simulink model "cichbcic_core"  (Simulink 7.9)
settings: Solver=ode45  StartTime=0.0  StopTime=10.0  RelTol=1e-3
libraries: xbsIndex_r4 x375
(part 1 of 5)
settings Model: Creator=chenhong  LastModifiedBy=chenhong

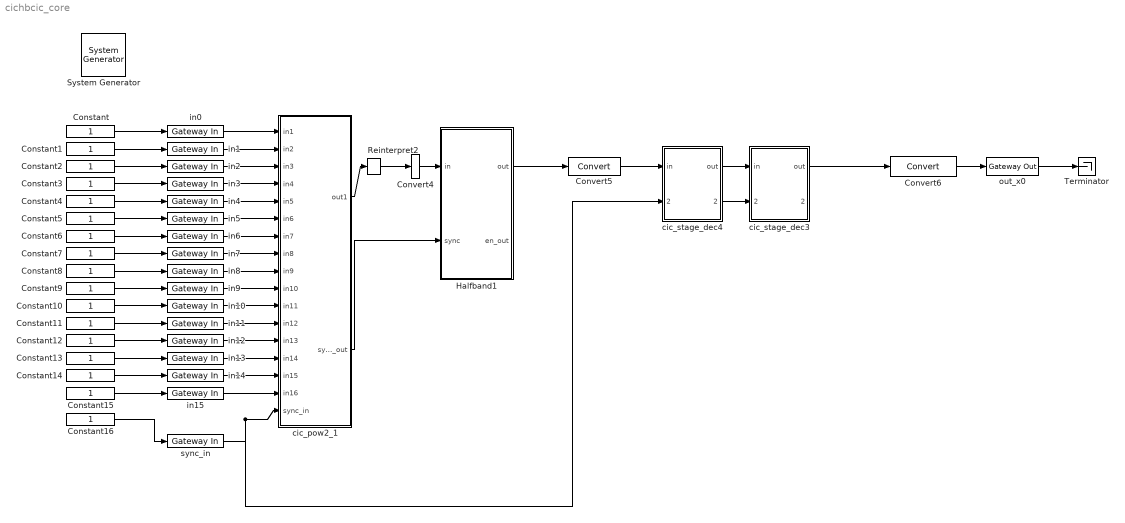
== system cichbcic_core ==
  " System Generator" : xbsIndex_r4/ System Generator  Tag=genX  xilinxfamily=virtex6  part=xc6vsx475t  speed=-1  package=ff1759  synthesis_tool=XST  clock_wrapper=Clock Enables  directory=./cichbcic_core  proj_type=Project Navigator  Synth_file=XST Defaults  Impl_file=ISE Defaults  testbench=off  simulink_period=1  sysclk_period=6.6667  dcm_input_clock_period=100  incr_netlist=off  trim_vbits=Everywhere in SubSystem  dbl_ovrd=According to Block Masks  core_generation=According to Block Masks  run_coregen=off  deprecated_control=off  eval_field=0  block_type=sysgen
  Constant{,1..16} (17 alike) : Constant
  Convert4 : xbsIndex_r4/Convert  gui_display_data_type=Fixed-point  arith_type="Signed  (2's comp)"  n_bits=32  bin_pt=18  float_type=Single  exp_bits=8  fraction_bits=24  quantization=Truncate  overflow=Wrap  en=off  latency=1  dbl_ovrd=off  pipeline=off  block_type=convert
  Convert5 : xbsIndex_r4/Convert  gui_display_data_type=Fixed-point  arith_type="Signed  (2's comp)"  n_bits=32  bin_pt=12  float_type=Single  exp_bits=8  fraction_bits=24  quantization=Truncate  overflow=Wrap  en=off  latency=1  dbl_ovrd=off  pipeline=off  block_type=convert
  Convert6 : xbsIndex_r4/Convert  gui_display_data_type=Fixed-point  arith_type="Signed  (2's comp)"  n_bits=32  bin_pt=6  float_type=Single  exp_bits=8  fraction_bits=24  quantization=Truncate  overflow=Wrap  en=off  latency=1  dbl_ovrd=off  pipeline=off  block_type=convert
  Halfband1 : Subsystem  AncestorBlock=gbt_library/Halfband  mask(Halfband FIR){mult_latency=3, add_latency=2, hold_period=2, passband=0.4, fir_len=7}
      mask prompts: mult_latency "Multiplication latency"; add_latency "Add latency"; hold_period "Hold Period"; passband "Width of Halfband passband (<0.5)"; fir_len "FIR Length (odd) [Number of Taps will be: 2*fir_len+1]"
      mask help: A halfband FIR for low rate computation.
      mask init:
      | coeffs = halfband_coeff_gen(fir_len, passband);
      | config.source=str2func('hold_fir_init_xblock');
      | config.depend=[get_dependlist('hold_fir'),{'halfband_coeff_gen'}];
      | config.toplevel=gcb;
      | set_param(gcb,'LinkStatus','inactive');
      | xBlock(config, {config.toplevel,...
      |     'mult_latency', mult_latency, ...
      |     'add_latency', add_latency, ...
      |     'hold_period', hold_period, ...
      |     'coeffs', coeffs});
      settings: AttributesFormatString=|
      | 15-tap FIR filter (9 nonzero tap)
      |  hold period: 2
      |  mult latency: 3
      |  add latency: 2
  Reinterpret2 : xbsIndex_r4/Reinterpret  force_arith_type=off  arith_type="Signed  (2's comp)"  force_bin_pt=on  bin_pt=30  block_type=reinterpret
  Terminator : Terminator
  cic_pow2_1 : Subsystem  AncestorBlock=gbt_library/cic_pow2  mask(CIC (pow2)){n_stages=4, dec_rate=32, input_clk_period=1, n_inputs=16, add_latency=1, n_bits=24, bin_pt=22}
      mask prompts: n_stages "CIC filter Order"; dec_rate "Decimation rate"; input_clk_period "Input Clock Period"; n_inputs "Number of inputs"; add_latency "Add latency"; n_bits "Input bit width"; bin_pt "Binary point"
      mask help:
      | A non-recursive CIC filter with parallel inputs.
      | Supports decimation rate of power of 2.
      | A multi-stage implementation with each stage of decimation rate 2.
      mask init:
      | config.source = str2func('cic_pow2_init_xblock');
      | config.toplevel = gcb;
      | config.depend = get_dependlist('cic_pow2'); 
      | set_param(gcb,'LinkStatus','inactive');
      | xBlock(config, {config.toplevel,...
      |                 'n_stages',n_stages, ...
      |                 'dec_rate', dec_rate, ...
      |                 'input_clk_rate', input_clk_period, ...
      |                 'n_inputs', n_inputs,...
      |                 'add_latency',add_latency,...
      |                 'n_bits', n_bits, ...
      |                 'bin_pt', bin_pt} ...
      |                 );
      | disp('new block added');
      settings: AttributesFormatString=|
      | dec_rate = 32
      | Order = 4
  cic_stage_dec3 : Subsystem  AncestorBlock=gbt_library/cic_stage_dec2  mask(CIC stage (dec2)){n_stages=3, recursive=off, dec_rate=2, n_inputs=1, input_clk_period=1, input_period=4, add_latency=2, n_bits=35, bin_pt=12}
      mask prompts: n_stages "CIC filter Order"; recursive "Recursive?"; dec_rate "Decimation rate"; n_inputs "Number of Inputs"; input_clk_period "Input Clock period (Actual)"; input_period "Effective Input Sampling Period"; add_latency "Add latency"; n_bits "Input bit width"; bin_pt "Binary point"
      mask help:
      | A single stage of CIC filter with even number of parallel inputs.
      | Only supports decimation rate = 2.
      | If n_inputs > 1, number of outputs = n_inputs/2.
      | Non-recursive.
      |
      | Clock period:
      | input_clk_period is the actual sampling period of incoming data stream.
      | input_period is the effective (or expected) sampling period of incoming data stream.
      | E.g. For incoming data stream X[n] = [1& 1 2 2 3 3 4 4 5 5 ...], the input_clk_period is 1 and the input_period is 2.
      mask init:
      | if recursive
      |     % recursive case
      |     config.source=str2func('cic_stage_dec2_recursive_init_xblock');
      |     config.toplevel=gcb;
      |     config.depend = get_dependlist('cic_stage_dec2_recursive');
      |     set_param(gcb,'LinkStatus','inactive');
      |     xBlock(config, {config.toplevel, ...
      |                 'n_stages', n_stages, ...
      |                 'dec_rate', dec_rate, ...
      |                 'n_inputs', n_inputs, ...
      |                 'input_clk_period', input_clk_period, ...
      |                 'input_period', input_period, ...
      |                 'add_latency', add_latency, ...
      |                 'input_bits', n_bits, ...
      |                 'bin_pt', bin_pt, ...
      |                 'delay_len', 1});
      | else
      |     % non-recursive case
      |     config.source=str2func('cic_stage_dec2_init_xblock');
      |     config.toplevel=gcb;
      |     config.depend = get_dependlist('cic_stage_dec2');
      |     set_param(gcb,'LinkStatus','inactive');
      |     xBlock(config, {config.toplevel, ...
      |                 'n_stages', n_stages, ...
      |                 'dec_rate', dec_rate, ...
      |                 'n_inputs', n_inputs, ...
      |                 'input_clk_period', input_clk_period, ...
      |                 'input_period', input_period, ...
      |                 'add_latency', add_latency, ...
      |                 'n_bits', n_bits, ...
      |                 'bin_pt', bin_pt});
      | end
      settings: AttributesFormatString=|
      | nonrecursive
      | 35_12_in
      | clock(actualy/effective): 1/4
      mask CallbackString:
      | ||n=get_param(gcb,'dec_rate');
      | if ~isempty(n)
      |     n = eval(n);
      |     if ~isprime(n) && n~=1
      |         errordlg('Only supports decimation rate that is a prime number or 1');
      |         set_param(gcb,'dec_rate','');
      |     end
      | end||||||
  cic_stage_dec4 : Subsystem  AncestorBlock=gbt_library/cic_stage_dec2  mask(CIC stage (dec2)){n_stages=3, recursive=off, dec_rate=2, n_inputs=1, input_clk_period=1, input_period=2, add_latency=2, n_bits=32, bin_pt=12}
      mask prompts: n_stages "CIC filter Order"; recursive "Recursive?"; dec_rate "Decimation rate"; n_inputs "Number of Inputs"; input_clk_period "Input Clock period (Actual)"; input_period "Effective Input Sampling Period"; add_latency "Add latency"; n_bits "Input bit width"; bin_pt "Binary point"
      mask help:
      | A single stage of CIC filter with even number of parallel inputs.
      | Only supports decimation rate = 2.
      | If n_inputs > 1, number of outputs = n_inputs/2.
      | Non-recursive.
      |
      | Clock period:
      | input_clk_period is the actual sampling period of incoming data stream.
      | input_period is the effective (or expected) sampling period of incoming data stream.
      | E.g. For incoming data stream X[n] = [1& 1 2 2 3 3 4 4 5 5 ...], the input_clk_period is 1 and the input_period is 2.
      mask init: same as cichbcic_core/cic_stage_dec3
      settings: AttributesFormatString=|
      | nonrecursive
      | 32_12_in
      | clock(actualy/effective): 1/2
      mask CallbackString:
      | ||n=get_param(gcb,'dec_rate');
      | if ~isempty(n)
      |     n = eval(n);
      |     if ~isprime(n) && n~=1
      |         errordlg('Only supports decimation rate that is a prime number or 1');
      |         set_param(gcb,'dec_rate','');
      |     end
      | end||||||
  in{0..15} (16 alike) : xbsIndex_r4/Gateway In  gui_display_data_type=Fixed-point  arith_type="Signed  (2's comp)"  n_bits=24  bin_pt=22  preci_type=Single  exp_width=8  frac_width=24  quantization="Round  (unbiased: +/- Inf)"  overflow=Saturate  period=1  dbl_ovrd=off  timing_constraint=None  locs_specified=off  LOCs={}  UseAsADC=off  ADCChannel='1'  inherit_from_input=off  hdl_port=on  block_type=gatewayin
  out_x0 : xbsIndex_r4/Gateway Out  inherit_from_input=off  hdl_port=on  timing_constraint=None  locs_specified=off  LOCs={}  UseAsDAC=off  DACChannel='1'  block_type=gatewayout
  sync_in : xbsIndex_r4/Gateway In  gui_display_data_type=Boolean  arith_type=Boolean  n_bits=24  bin_pt=22  preci_type=Single  exp_width=8  frac_width=24  quantization="Round  (unbiased: +/- Inf)"  overflow=Saturate  period=1  dbl_ovrd=off  timing_constraint=None  locs_specified=off  LOCs={}  UseAsADC=off  ADCChannel='1'  inherit_from_input=off  hdl_port=on  block_type=gatewayin
  wires:
  cic_stage_dec4/2(sync_out) -> cic_stage_dec3/2(sync_in)
  cic_stage_dec4/1(out) -> cic_stage_dec3/1(in)
  Halfband1/1(out) -> Convert5/1
  cic_pow2_1/1(out1) -> Reinterpret2/1
  cic_pow2_1/2(sync_out) -> Halfband1/2(sync)
  Convert4/1 -> Halfband1/1(in)
  Convert5/1 -> cic_stage_dec4/1(in)
  Convert6/1 -> out_x0/1
  cic_stage_dec3/1(out) -> Convert6/1
  Reinterpret2/1 -> Convert4/1
  in0/1 -> cic_pow2_1/1(in1)
  in1/1 -> cic_pow2_1/2(in2)
  in2/1 -> cic_pow2_1/3(in3)
  in3/1 -> cic_pow2_1/4(in4)
  in4/1 -> cic_pow2_1/5(in5)
  in5/1 -> cic_pow2_1/6(in6)
  in6/1 -> cic_pow2_1/7(in7)
  in7/1 -> cic_pow2_1/8(in8)
  in8/1 -> cic_pow2_1/9(in9)
  in9/1 -> cic_pow2_1/10(in10)
  in10/1 -> cic_pow2_1/11(in11)
  in11/1 -> cic_pow2_1/12(in12)
  in12/1 -> cic_pow2_1/13(in13)
  in13/1 -> cic_pow2_1/14(in14)
  in14/1 -> cic_pow2_1/15(in15)
  in15/1 -> cic_pow2_1/16(in16)
  sync_in/1 -> cic_pow2_1/17(sync_in), cic_stage_dec4/2(sync_in)
  Constant/1 -> in0/1
  Constant1/1 -> in1/1
  Constant2/1 -> in2/1
  Constant3/1 -> in3/1
  Constant4/1 -> in4/1
  Constant5/1 -> in5/1
  Constant6/1 -> in6/1
  Constant7/1 -> in7/1
  Constant8/1 -> in8/1
  Constant9/1 -> in9/1
  Constant10/1 -> in10/1
  Constant11/1 -> in11/1
  Constant12/1 -> in12/1
  Constant13/1 -> in13/1
  Constant14/1 -> in14/1
  Constant15/1 -> in15/1
  Constant16/1 -> sync_in/1
  out_x0/1 -> Terminator/1

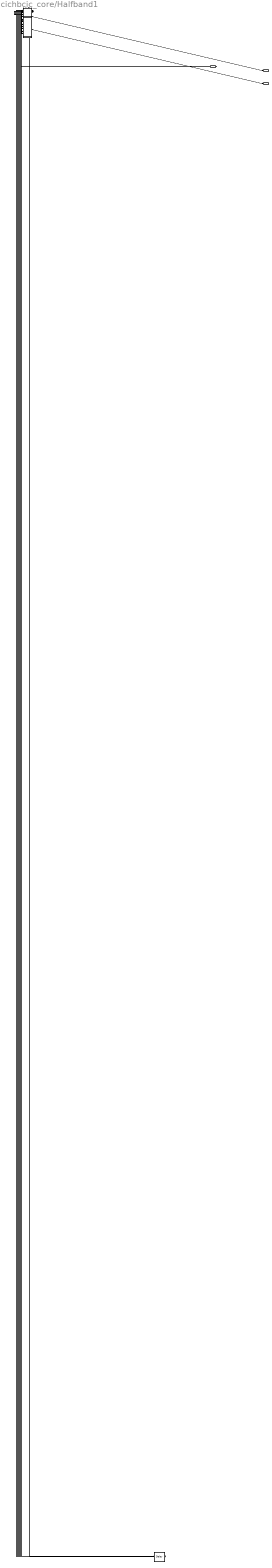
== system cichbcic_core/Halfband1 ==
  in : Inport
  sync : Inport  Port=2
  Delay{1..14} (14 alike) : xbsIndex_r4/Delay  rst=off  infoeditControl=Selection of Reset will increase slice count due to use of real FFs and instead of SRLs  en=off  latency=2  dbl_ovrd=off  reg_retiming=off  block_type=delay
  adder_tree : Subsystem
      settings: AttributesFormatString=|
      | latency 8
      | hold period:2
  en_gen : Subsystem
      settings: AttributesFormatString=|
      | hold period: 2
      | explicit clk period:off , input clk period:1
  hold_fir_tap1 : Subsystem
      settings: AttributesFormatString=|
      | coefficient: -0.026473
      |  hold period: 2
      |  mult latency: 3
  hold_fir_tap11 : Subsystem
      settings: AttributesFormatString=|
      | coefficient: -0.093407
      |  hold period: 2
      |  mult latency: 3
  hold_fir_tap13 : Subsystem
      settings: AttributesFormatString=|
      | coefficient: 0.044090
      |  hold period: 2
      |  mult latency: 3
  hold_fir_tap15 : Subsystem
      settings: AttributesFormatString=|
      | coefficient: -0.026473
      |  hold period: 2
      |  mult latency: 3
  hold_fir_tap3 : Subsystem
      settings: AttributesFormatString=|
      | coefficient: 0.044090
      |  hold period: 2
      |  mult latency: 3
  hold_fir_tap5 : Subsystem
      settings: AttributesFormatString=|
      | coefficient: -0.093407
      |  hold period: 2
      |  mult latency: 3
  hold_fir_tap7 : Subsystem
      settings: AttributesFormatString=|
      | coefficient: 0.313910
      |  hold period: 2
      |  mult latency: 3
  hold_fir_tap8 : Subsystem
      settings: AttributesFormatString=|
      | coefficient: 0.500000
      |  hold period: 2
      |  mult latency: 3
  hold_fir_tap9 : Subsystem
      settings: AttributesFormatString=|
      | coefficient: 0.313910
      |  hold period: 2
      |  mult latency: 3
  out : Outport
  en_out : Outport  Port=2
  wires:
  sync/1 -> en_gen/1(sync_in)
  in/1 -> Delay1/1, hold_fir_tap1/1(data_in)
  Delay1/1 -> Delay2/1  "xlsub2_Delay_out1"
  Delay2/1 -> Delay3/1, hold_fir_tap3/1(data_in)  "xlsub2_Delay_out2"
  Delay3/1 -> Delay4/1  "xlsub2_Delay_out3"
  Delay4/1 -> Delay5/1, hold_fir_tap5/1(data_in)  "xlsub2_Delay_out4"
  Delay5/1 -> Delay6/1  "xlsub2_Delay_out5"
  Delay6/1 -> Delay7/1, hold_fir_tap7/1(data_in)  "xlsub2_Delay_out6"
  Delay7/1 -> Delay8/1, hold_fir_tap8/1(data_in)  "xlsub2_Delay_out7"
  Delay8/1 -> Delay9/1, hold_fir_tap9/1(data_in)  "xlsub2_Delay_out8"
  Delay9/1 -> Delay10/1  "xlsub2_Delay_out9"
  Delay10/1 -> Delay11/1, hold_fir_tap11/1(data_in)  "xlsub2_Delay_out10"
  Delay11/1 -> Delay12/1  "xlsub2_Delay_out11"
  Delay12/1 -> Delay13/1, hold_fir_tap13/1(data_in)  "xlsub2_Delay_out12"
  Delay13/1 -> Delay14/1  "xlsub2_Delay_out13"
  en_gen/1(en_out) -> hold_fir_tap1/2(en_in), hold_fir_tap3/2(en_in), hold_fir_tap5/2(en_in), hold_fir_tap7/2(en_in), hold_fir_tap8/2(en_in), hold_fir_tap9/2(en_in), hold_fir_tap11/2(en_in), hold_fir_tap13/2(en_in), hold_fir_tap15/2(en_in), adder_tree/1(en_in)  "en"
  Delay14/1 -> hold_fir_tap15/1(data_in)  "xlsub2_Delay_out14"
  hold_fir_tap1/1(mult_out) -> adder_tree/2(din1)  "hold_fir_tap_out1"
  hold_fir_tap3/1(mult_out) -> adder_tree/3(din2)  "hold_fir_tap_out2"
  hold_fir_tap5/1(mult_out) -> adder_tree/4(din3)  "hold_fir_tap_out3"
  hold_fir_tap7/1(mult_out) -> adder_tree/5(din4)  "hold_fir_tap_out4"
  hold_fir_tap8/1(mult_out) -> adder_tree/6(din5)  "hold_fir_tap_out5"
  hold_fir_tap9/1(mult_out) -> adder_tree/7(din6)  "hold_fir_tap_out6"
  hold_fir_tap11/1(mult_out) -> adder_tree/8(din7)  "hold_fir_tap_out7"
  hold_fir_tap13/1(mult_out) -> adder_tree/9(din8)  "hold_fir_tap_out8"
  hold_fir_tap15/1(mult_out) -> adder_tree/10(din9)  "hold_fir_tap_out9"
  adder_tree/1(en_out) -> en_out/1
  adder_tree/2(dout) -> out/1

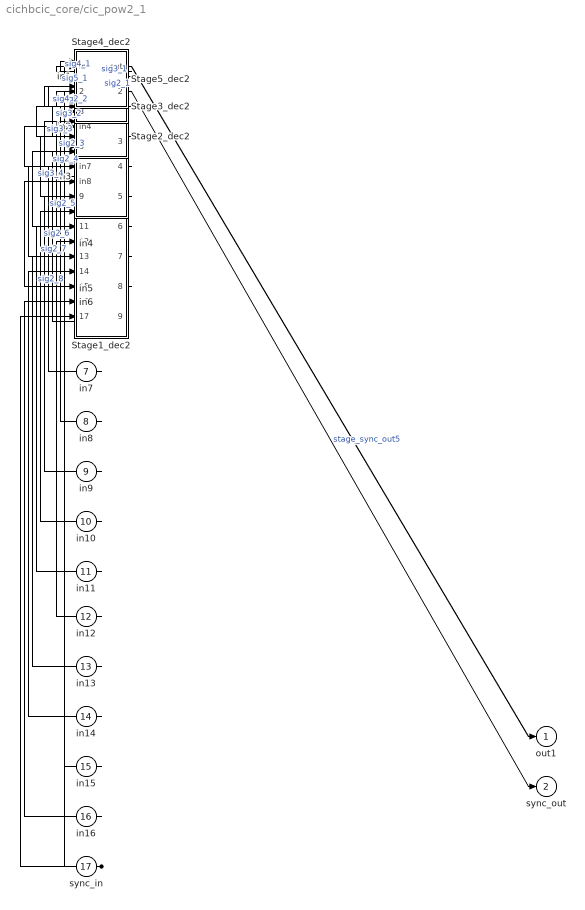
== system cichbcic_core/cic_pow2_1 ==
  in1 : Inport
  in2 : Inport  Port=2
  in3 : Inport  Port=3
  in4 : Inport  Port=4
  in5 : Inport  Port=5
  in6 : Inport  Port=6
  in7 : Inport  Port=7
  in8 : Inport  Port=8
  in9 : Inport  Port=9
  in10 : Inport  Port=10
  in11 : Inport  Port=11
  in12 : Inport  Port=12
  in13 : Inport  Port=13
  in14 : Inport  Port=14
  in15 : Inport  Port=15
  in16 : Inport  Port=16
  sync_in : Inport  Port=17
  Stage1_dec2 : Subsystem
      settings: AttributesFormatString=|
      | nonrecursive
      | 24_22_in
      | clock(actualy/effective): 1/1
  Stage2_dec2 : Subsystem
      settings: AttributesFormatString=|
      | nonrecursive
      | 28_22_in
      | clock(actualy/effective): 1/1
  Stage3_dec2 : Subsystem
      settings: AttributesFormatString=|
      | nonrecursive
      | 32_22_in
      | clock(actualy/effective): 1/1
  Stage4_dec2 : Subsystem
      settings: AttributesFormatString=|
      | nonrecursive
      | 36_22_in
      | clock(actualy/effective): 1/1
  Stage5_dec2 : Subsystem
      settings: AttributesFormatString=|
      | nonrecursive
      | 40_22_in
      | clock(actualy/effective): 1/1
  out1 : Outport
  sync_out : Outport  Port=2
  wires:
  in1/1 -> Stage1_dec2/1(in1)
  in2/1 -> Stage1_dec2/2(in2)
  in3/1 -> Stage1_dec2/3(in3)
  in4/1 -> Stage1_dec2/4(in4)
  in5/1 -> Stage1_dec2/5(in5)
  in6/1 -> Stage1_dec2/6(in6)
  in7/1 -> Stage1_dec2/7(in7)
  in8/1 -> Stage1_dec2/8(in8)
  in9/1 -> Stage1_dec2/9(in9)
  in10/1 -> Stage1_dec2/10(in10)
  in11/1 -> Stage1_dec2/11(in11)
  in12/1 -> Stage1_dec2/12(in12)
  in13/1 -> Stage1_dec2/13(in13)
  in14/1 -> Stage1_dec2/14(in14)
  in15/1 -> Stage1_dec2/15(in15)
  in16/1 -> Stage1_dec2/16(in16)
  sync_in/1 -> Stage1_dec2/17(sync_in), Stage2_dec2/9(sync_in), Stage3_dec2/5(sync_in), Stage4_dec2/3(sync_in), Stage5_dec2/2(sync_in)
  Stage1_dec2/1(out1) -> Stage2_dec2/1(in1)  "sig2_1"
  Stage1_dec2/2(out2) -> Stage2_dec2/2(in2)  "sig2_2"
  Stage1_dec2/3(out3) -> Stage2_dec2/3(in3)  "sig2_3"
  Stage1_dec2/4(out4) -> Stage2_dec2/4(in4)  "sig2_4"
  Stage1_dec2/5(out5) -> Stage2_dec2/5(in5)  "sig2_5"
  Stage1_dec2/6(out6) -> Stage2_dec2/6(in6)  "sig2_6"
  Stage1_dec2/7(out7) -> Stage2_dec2/7(in7)  "sig2_7"
  Stage1_dec2/8(out8) -> Stage2_dec2/8(in8)  "sig2_8"
  Stage2_dec2/1(out1) -> Stage3_dec2/1(in1)  "sig3_1"
  Stage2_dec2/2(out2) -> Stage3_dec2/2(in2)  "sig3_2"
  Stage2_dec2/3(out3) -> Stage3_dec2/3(in3)  "sig3_3"
  Stage2_dec2/4(out4) -> Stage3_dec2/4(in4)  "sig3_4"
  Stage3_dec2/1(out1) -> Stage4_dec2/1(in1)  "sig4_1"
  Stage3_dec2/2(out2) -> Stage4_dec2/2(in2)  "sig4_2"
  Stage4_dec2/1(out1) -> Stage5_dec2/1(in)  "sig5_1"
  Stage5_dec2/1(out) -> out1/1
  Stage5_dec2/2(sync_out) -> sync_out/1  "stage_sync_out5"

== system cichbcic_core/cic_stage_dec3 ==
  in : Inport
  sync_in : Inport  Port=2
  Down_sample1 : Subsystem
      settings: AttributesFormatString=|
      | Rate change: 2
      | clock(actualy/effective): 1/4
  adder_tree1 : Subsystem
  adder_tree2 : Subsystem
  adder_tree3 : Subsystem
  delay1_1 : xbsIndex_r4/Delay  rst=off  infoeditControl=Selection of Reset will increase slice count due to use of real FFs and instead of SRLs  en=off  latency=4  dbl_ovrd=off  reg_retiming=off  block_type=delay
  delay2_1 : xbsIndex_r4/Delay  rst=off  infoeditControl=Selection of Reset will increase slice count due to use of real FFs and instead of SRLs  en=off  latency=4  dbl_ovrd=off  reg_retiming=off  block_type=delay
  delay3_1 : xbsIndex_r4/Delay  rst=off  infoeditControl=Selection of Reset will increase slice count due to use of real FFs and instead of SRLs  en=off  latency=4  dbl_ovrd=off  reg_retiming=off  block_type=delay
  out : Outport
  sync_out : Outport  Port=2
  wires:
  in/1 -> delay1_1/1, adder_tree1/1(sync), adder_tree1/2(din_1)
  delay1_1/1 -> adder_tree1/3(din_2)  "delay_out1_2"
  adder_tree1/2(dout) -> delay2_1/1, adder_tree2/2(din_1)  "delay_in1_1"
  adder_tree1/1(sync_out) -> adder_tree2/1(sync)  "adder_tree_sync_in2"
  delay2_1/1 -> adder_tree2/3(din_2)  "delay_out2_2"
  adder_tree2/2(dout) -> delay3_1/1, adder_tree3/2(din_1)  "delay_in2_1"
  adder_tree2/1(sync_out) -> adder_tree3/1(sync)  "adder_tree_sync_in3"
  delay3_1/1 -> adder_tree3/3(din_2)  "delay_out3_2"
  adder_tree3/2(dout) -> Down_sample1/1(In)  "delay_in3_1"
  sync_in/1 -> Down_sample1/2(sync_in)
  Down_sample1/1(Out) -> out/1
  Down_sample1/2(sync_out) -> sync_out/1

== system cichbcic_core/cic_stage_dec4 ==
  in : Inport
  sync_in : Inport  Port=2
  Down_sample1 : Subsystem
      settings: AttributesFormatString=|
      | Rate change: 2
      | clock(actualy/effective): 1/2
  adder_tree1 : Subsystem
  adder_tree2 : Subsystem
  adder_tree3 : Subsystem
  delay1_1 : xbsIndex_r4/Delay  rst=off  infoeditControl=Selection of Reset will increase slice count due to use of real FFs and instead of SRLs  en=off  latency=2  dbl_ovrd=off  reg_retiming=off  block_type=delay
  delay2_1 : xbsIndex_r4/Delay  rst=off  infoeditControl=Selection of Reset will increase slice count due to use of real FFs and instead of SRLs  en=off  latency=2  dbl_ovrd=off  reg_retiming=off  block_type=delay
  delay3_1 : xbsIndex_r4/Delay  rst=off  infoeditControl=Selection of Reset will increase slice count due to use of real FFs and instead of SRLs  en=off  latency=2  dbl_ovrd=off  reg_retiming=off  block_type=delay
  out : Outport
  sync_out : Outport  Port=2
  wires:
  in/1 -> delay1_1/1, adder_tree1/1(sync), adder_tree1/2(din_1)
  delay1_1/1 -> adder_tree1/3(din_2)  "delay_out1_2"
  adder_tree1/2(dout) -> delay2_1/1, adder_tree2/2(din_1)  "delay_in1_1"
  adder_tree1/1(sync_out) -> adder_tree2/1(sync)  "adder_tree_sync_in2"
  delay2_1/1 -> adder_tree2/3(din_2)  "delay_out2_2"
  adder_tree2/2(dout) -> delay3_1/1, adder_tree3/2(din_1)  "delay_in2_1"
  adder_tree2/1(sync_out) -> adder_tree3/1(sync)  "adder_tree_sync_in3"
  delay3_1/1 -> adder_tree3/3(din_2)  "delay_out3_2"
  adder_tree3/2(dout) -> Down_sample1/1(In)  "delay_in3_1"
  sync_in/1 -> Down_sample1/2(sync_in)
  Down_sample1/1(Out) -> out/1
  Down_sample1/2(sync_out) -> sync_out/1

== system cichbcic_core/Halfband1/adder_tree ==
  en_in : Inport
  din1 : Inport  Port=2
  din2 : Inport  Port=3
  din3 : Inport  Port=4
  din4 : Inport  Port=5
  din5 : Inport  Port=6
  din6 : Inport  Port=7
  din7 : Inport  Port=8
  din8 : Inport  Port=9
  din9 : Inport  Port=10
  addr1 : Subsystem
      settings: AttributesFormatString=|
      | hold period: 2
      |  add latency: 2
  addr11 : Subsystem
      settings: AttributesFormatString=|
      | hold period: 2
      |  add latency: 2
  addr2 : Subsystem
      settings: AttributesFormatString=|
      | hold period: 2
      |  add latency: 2
  addr3 : Subsystem
      settings: AttributesFormatString=|
      | hold period: 2
      |  add latency: 2
  addr4 : Subsystem
      settings: AttributesFormatString=|
      | hold period: 2
      |  add latency: 2
  addr6 : Subsystem
      settings: AttributesFormatString=|
      | hold period: 2
      |  add latency: 2
  addr7 : Subsystem
      settings: AttributesFormatString=|
      | hold period: 2
      |  add latency: 2
  addr9 : Subsystem
      settings: AttributesFormatString=|
      | hold period: 2
      |  add latency: 2
  dly10 : xbsIndex_r4/Delay  rst=off  infoeditControl=Selection of Reset will increase slice count due to use of real FFs and instead of SRLs  en=off  latency=4  dbl_ovrd=off  reg_retiming=on  block_type=delay
  dly5 : xbsIndex_r4/Delay  rst=off  infoeditControl=Selection of Reset will increase slice count due to use of real FFs and instead of SRLs  en=off  latency=4  dbl_ovrd=off  reg_retiming=on  block_type=delay
  dly8 : xbsIndex_r4/Delay  rst=off  infoeditControl=Selection of Reset will increase slice count due to use of real FFs and instead of SRLs  en=off  latency=4  dbl_ovrd=off  reg_retiming=on  block_type=delay
  sync_delay : xbsIndex_r4/Delay  rst=off  infoeditControl=Selection of Reset will increase slice count due to use of real FFs and instead of SRLs  en=off  latency=8  dbl_ovrd=off  reg_retiming=on  block_type=delay
  en_out : Outport
  dout : Outport  Port=2
  wires:
  en_in/1 -> sync_delay/1, addr1/3(en_in), addr2/3(en_in), addr3/3(en_in), addr4/3(en_in), addr6/3(en_in), addr7/3(en_in), addr9/3(en_in), addr11/3(en_in)
  sync_delay/1 -> en_out/1
  din1/1 -> addr1/1(data_a)
  din2/1 -> addr1/2(data_b)
  din3/1 -> addr2/1(data_a)
  din4/1 -> addr2/2(data_b)
  din5/1 -> addr3/1(data_a)
  din6/1 -> addr3/2(data_b)
  din7/1 -> addr4/1(data_a)
  din8/1 -> addr4/2(data_b)
  din9/1 -> dly5/1
  addr1/1(sum_ab) -> addr6/1(data_a)  "adder_outs1_1"
  addr2/1(sum_ab) -> addr6/2(data_b)  "adder_outs1_2"
  addr3/1(sum_ab) -> addr7/1(data_a)  "adder_outs1_3"
  addr4/1(sum_ab) -> addr7/2(data_b)  "adder_outs1_4"
  dly5/1 -> dly8/1  "adder_outs1_5"
  addr6/1(sum_ab) -> addr9/1(data_a)  "adder_outs2_1"
  addr7/1(sum_ab) -> addr9/2(data_b)  "adder_outs2_2"
  dly8/1 -> dly10/1  "adder_outs2_3"
  addr9/1(sum_ab) -> addr11/1(data_a)  "adder_outs3_1"
  dly10/1 -> addr11/2(data_b)  "adder_outs3_2"
  addr11/1(sum_ab) -> dout/1  "adder_outs4_1"

== system cichbcic_core/Halfband1/en_gen ==
  sync_in : Inport
  Constant : xbsIndex_r4/Constant  const=0  gui_display_data_type=Fixed-point  arith_type=Signed (2's comp)  n_bits=16  bin_pt=14  preci_type=Single  exp_width=8  frac_width=24  explicit_period=off  period=1  equ=P=C  opselect=C  inp2=PCIN>>17  opr=+  inp1=P  carry=CIN  dbl_ovrd=off  block_type=constant
  Counter1 : xbsIndex_r4/Counter  cnt_type=Count Limited  cnt_to=0  operation=Down  start_count=1  cnt_by_val=1  arith_type=Unsigned  n_bits=1  bin_pt=0  load_pin=off  rst=on  en=off  explicit_period=on  period=1  dbl_ovrd=off  use_behavioral_HDL=off  implementation=Fabric  block_type=counter
  Logical : xbsIndex_r4/Logical  logical_function=OR  inputs=2  en=off  latency=0  precision=Full  arith_type=Unsigned  n_bits=16  bin_pt=0  align_bp=on  dbl_ovrd=off  block_type=logical
  Relational : xbsIndex_r4/Relational  mode=a=b  en=off  latency=0  dbl_ovrd=off  block_type=relational
  en_out : Outport
  wires:
  sync_in/1 -> Logical/2
  Logical/1 -> Counter1/1, en_out/1  "xlsub1_Logical_out1"
  Counter1/1 -> Relational/1  "xlsub1_Counter1_out1"
  Constant/1 -> Relational/2  "xlsub1_Constant_out1"
  Relational/1 -> Logical/1  "xlsub1_Relational_out1"

== system cichbcic_core/Halfband1/hold_fir_tap1 ==
  data_in : Inport
  en_in : Inport  Port=2
  Mult : xbsIndex_r4/Mult  precision=Full  arith_type="Signed  (2's comp)"  n_bits=16  bin_pt=14  quantization=Truncate  overflow=Wrap  en=on  latency=3  dbl_ovrd=off  use_behavioral_HDL=off  opt=Speed  use_embedded=on  optimum_pipeline=off  pipeline=on  use_rpm=on  placement_style=Triangular  block_type=mult
  coefficient : xbsIndex_r4/Constant  const=-0.026472867764434  gui_display_data_type=Fixed-point  arith_type=Signed (2's comp)  n_bits=16  bin_pt=14  preci_type=Single  exp_width=8  frac_width=24  explicit_period=on  period=1  equ=P=C  opselect=C  inp2=PCIN>>17  opr=+  inp1=P  carry=CIN  dbl_ovrd=off  block_type=constant
  mult_out : Outport
  en_out : Outport  Port=2
  wires:
  data_in/1 -> Mult/2
  en_in/1 -> Mult/3, en_out/1
  Mult/1 -> mult_out/1
  coefficient/1 -> Mult/1  "xlsub2_coefficient_out1"

== system cichbcic_core/Halfband1/hold_fir_tap11 ==
  data_in : Inport
  en_in : Inport  Port=2
  Mult : xbsIndex_r4/Mult  precision=Full  arith_type="Signed  (2's comp)"  n_bits=16  bin_pt=14  quantization=Truncate  overflow=Wrap  en=on  latency=3  dbl_ovrd=off  use_behavioral_HDL=off  opt=Speed  use_embedded=on  optimum_pipeline=off  pipeline=on  use_rpm=on  placement_style=Triangular  block_type=mult
  coefficient : xbsIndex_r4/Constant  const=-0.0934071809736732  gui_display_data_type=Fixed-point  arith_type=Signed (2's comp)  n_bits=16  bin_pt=14  preci_type=Single  exp_width=8  frac_width=24  explicit_period=on  period=1  equ=P=C  opselect=C  inp2=PCIN>>17  opr=+  inp1=P  carry=CIN  dbl_ovrd=off  block_type=constant
  mult_out : Outport
  en_out : Outport  Port=2
  wires:
  data_in/1 -> Mult/2
  en_in/1 -> Mult/3, en_out/1
  Mult/1 -> mult_out/1
  coefficient/1 -> Mult/1  "xlsub2_coefficient_out1"

== system cichbcic_core/Halfband1/hold_fir_tap13 ==
  data_in : Inport
  en_in : Inport  Port=2
  Mult : xbsIndex_r4/Mult  precision=Full  arith_type="Signed  (2's comp)"  n_bits=16  bin_pt=14  quantization=Truncate  overflow=Wrap  en=on  latency=3  dbl_ovrd=off  use_behavioral_HDL=off  opt=Speed  use_embedded=on  optimum_pipeline=off  pipeline=on  use_rpm=on  placement_style=Triangular  block_type=mult
  coefficient : xbsIndex_r4/Constant  const=0.0440903441068704  gui_display_data_type=Fixed-point  arith_type=Signed (2's comp)  n_bits=16  bin_pt=14  preci_type=Single  exp_width=8  frac_width=24  explicit_period=on  period=1  equ=P=C  opselect=C  inp2=PCIN>>17  opr=+  inp1=P  carry=CIN  dbl_ovrd=off  block_type=constant
  mult_out : Outport
  en_out : Outport  Port=2
  wires:
  data_in/1 -> Mult/2
  en_in/1 -> Mult/3, en_out/1
  Mult/1 -> mult_out/1
  coefficient/1 -> Mult/1  "xlsub2_coefficient_out1"

== system cichbcic_core/Halfband1/hold_fir_tap15 ==
  data_in : Inport
  en_in : Inport  Port=2
  Mult : xbsIndex_r4/Mult  precision=Full  arith_type="Signed  (2's comp)"  n_bits=16  bin_pt=14  quantization=Truncate  overflow=Wrap  en=on  latency=3  dbl_ovrd=off  use_behavioral_HDL=off  opt=Speed  use_embedded=on  optimum_pipeline=off  pipeline=on  use_rpm=on  placement_style=Triangular  block_type=mult
  coefficient : xbsIndex_r4/Constant  const=-0.026472867764434  gui_display_data_type=Fixed-point  arith_type=Signed (2's comp)  n_bits=16  bin_pt=14  preci_type=Single  exp_width=8  frac_width=24  explicit_period=on  period=1  equ=P=C  opselect=C  inp2=PCIN>>17  opr=+  inp1=P  carry=CIN  dbl_ovrd=off  block_type=constant
  mult_out : Outport
  en_out : Outport  Port=2
  wires:
  data_in/1 -> Mult/2
  en_in/1 -> Mult/3, en_out/1
  Mult/1 -> mult_out/1
  coefficient/1 -> Mult/1  "xlsub2_coefficient_out1"

== system cichbcic_core/Halfband1/hold_fir_tap3 ==
  data_in : Inport
  en_in : Inport  Port=2
  Mult : xbsIndex_r4/Mult  precision=Full  arith_type="Signed  (2's comp)"  n_bits=16  bin_pt=14  quantization=Truncate  overflow=Wrap  en=on  latency=3  dbl_ovrd=off  use_behavioral_HDL=off  opt=Speed  use_embedded=on  optimum_pipeline=off  pipeline=on  use_rpm=on  placement_style=Triangular  block_type=mult
  coefficient : xbsIndex_r4/Constant  const=0.0440903441068704  gui_display_data_type=Fixed-point  arith_type=Signed (2's comp)  n_bits=16  bin_pt=14  preci_type=Single  exp_width=8  frac_width=24  explicit_period=on  period=1  equ=P=C  opselect=C  inp2=PCIN>>17  opr=+  inp1=P  carry=CIN  dbl_ovrd=off  block_type=constant
  mult_out : Outport
  en_out : Outport  Port=2
  wires:
  data_in/1 -> Mult/2
  en_in/1 -> Mult/3, en_out/1
  Mult/1 -> mult_out/1
  coefficient/1 -> Mult/1  "xlsub2_coefficient_out1"

== system cichbcic_core/Halfband1/hold_fir_tap5 ==
  data_in : Inport
  en_in : Inport  Port=2
  Mult : xbsIndex_r4/Mult  precision=Full  arith_type="Signed  (2's comp)"  n_bits=16  bin_pt=14  quantization=Truncate  overflow=Wrap  en=on  latency=3  dbl_ovrd=off  use_behavioral_HDL=off  opt=Speed  use_embedded=on  optimum_pipeline=off  pipeline=on  use_rpm=on  placement_style=Triangular  block_type=mult
  coefficient : xbsIndex_r4/Constant  const=-0.0934071809736732  gui_display_data_type=Fixed-point  arith_type=Signed (2's comp)  n_bits=16  bin_pt=14  preci_type=Single  exp_width=8  frac_width=24  explicit_period=on  period=1  equ=P=C  opselect=C  inp2=PCIN>>17  opr=+  inp1=P  carry=CIN  dbl_ovrd=off  block_type=constant
  mult_out : Outport
  en_out : Outport  Port=2
  wires:
  data_in/1 -> Mult/2
  en_in/1 -> Mult/3, en_out/1
  Mult/1 -> mult_out/1
  coefficient/1 -> Mult/1  "xlsub2_coefficient_out1"

== system cichbcic_core/Halfband1/hold_fir_tap7 ==
  data_in : Inport
  en_in : Inport  Port=2
  Mult : xbsIndex_r4/Mult  precision=Full  arith_type="Signed  (2's comp)"  n_bits=16  bin_pt=14  quantization=Truncate  overflow=Wrap  en=on  latency=3  dbl_ovrd=off  use_behavioral_HDL=off  opt=Speed  use_embedded=on  optimum_pipeline=off  pipeline=on  use_rpm=on  placement_style=Triangular  block_type=mult
  coefficient : xbsIndex_r4/Constant  const=0.313910410160698  gui_display_data_type=Fixed-point  arith_type=Signed (2's comp)  n_bits=16  bin_pt=14  preci_type=Single  exp_width=8  frac_width=24  explicit_period=on  period=1  equ=P=C  opselect=C  inp2=PCIN>>17  opr=+  inp1=P  carry=CIN  dbl_ovrd=off  block_type=constant
  mult_out : Outport
  en_out : Outport  Port=2
  wires:
  data_in/1 -> Mult/2
  en_in/1 -> Mult/3, en_out/1
  Mult/1 -> mult_out/1
  coefficient/1 -> Mult/1  "xlsub2_coefficient_out1"

== system cichbcic_core/Halfband1/hold_fir_tap8 ==
  data_in : Inport
  en_in : Inport  Port=2
  Mult : xbsIndex_r4/Mult  precision=Full  arith_type="Signed  (2's comp)"  n_bits=16  bin_pt=14  quantization=Truncate  overflow=Wrap  en=on  latency=3  dbl_ovrd=off  use_behavioral_HDL=off  opt=Speed  use_embedded=on  optimum_pipeline=off  pipeline=on  use_rpm=on  placement_style=Triangular  block_type=mult
  coefficient : xbsIndex_r4/Constant  const=0.5  gui_display_data_type=Fixed-point  arith_type=Signed (2's comp)  n_bits=16  bin_pt=14  preci_type=Single  exp_width=8  frac_width=24  explicit_period=on  period=1  equ=P=C  opselect=C  inp2=PCIN>>17  opr=+  inp1=P  carry=CIN  dbl_ovrd=off  block_type=constant
  mult_out : Outport
  en_out : Outport  Port=2
  wires:
  data_in/1 -> Mult/2
  en_in/1 -> Mult/3, en_out/1
  Mult/1 -> mult_out/1
  coefficient/1 -> Mult/1  "xlsub2_coefficient_out1"

== system cichbcic_core/Halfband1/hold_fir_tap9 ==
  data_in : Inport
  en_in : Inport  Port=2
  Mult : xbsIndex_r4/Mult  precision=Full  arith_type="Signed  (2's comp)"  n_bits=16  bin_pt=14  quantization=Truncate  overflow=Wrap  en=on  latency=3  dbl_ovrd=off  use_behavioral_HDL=off  opt=Speed  use_embedded=on  optimum_pipeline=off  pipeline=on  use_rpm=on  placement_style=Triangular  block_type=mult
  coefficient : xbsIndex_r4/Constant  const=0.313910410160698  gui_display_data_type=Fixed-point  arith_type=Signed (2's comp)  n_bits=16  bin_pt=14  preci_type=Single  exp_width=8  frac_width=24  explicit_period=on  period=1  equ=P=C  opselect=C  inp2=PCIN>>17  opr=+  inp1=P  carry=CIN  dbl_ovrd=off  block_type=constant
  mult_out : Outport
  en_out : Outport  Port=2
  wires:
  data_in/1 -> Mult/2
  en_in/1 -> Mult/3, en_out/1
  Mult/1 -> mult_out/1
  coefficient/1 -> Mult/1  "xlsub2_coefficient_out1"

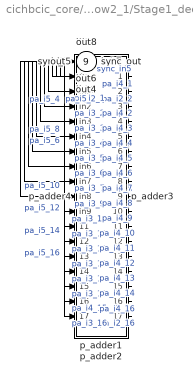
== system cichbcic_core/cic_pow2_1/Stage1_dec2 ==
  in1 : Inport
  in2 : Inport  Port=2
  in3 : Inport  Port=3
  in4 : Inport  Port=4
  in5 : Inport  Port=5
  in6 : Inport  Port=6
  in7 : Inport  Port=7
  in8 : Inport  Port=8
  in9 : Inport  Port=9
  in10 : Inport  Port=10
  in11 : Inport  Port=11
  in12 : Inport  Port=12
  in13 : Inport  Port=13
  in14 : Inport  Port=14
  in15 : Inport  Port=15
  in16 : Inport  Port=16
  sync_in : Inport  Port=17
  p_adder1 : Subsystem
      settings: AttributesFormatString=|
      | Accumulation Length = 2
      | Add Latency = 1
      | Delay Length =1
  p_adder2 : Subsystem
      settings: AttributesFormatString=|
      | Accumulation Length = 2
      | Add Latency = 1
      | Delay Length =1
  p_adder3 : Subsystem
      settings: AttributesFormatString=|
      | Accumulation Length = 2
      | Add Latency = 1
      | Delay Length =1
  p_adder4 : Subsystem
      settings: AttributesFormatString=|
      | Accumulation Length = 2
      | Add Latency = 1
      | Delay Length =1
  out1 : Outport
  out2 : Outport  Port=2
  out3 : Outport  Port=3
  out4 : Outport  Port=4
  out5 : Outport  Port=5
  out6 : Outport  Port=6
  out7 : Outport  Port=7
  out8 : Outport  Port=8
  sync_out : Outport  Port=9
  wires:
  sync_in/1 -> p_adder1/1(sync_in), p_adder2/1(sync_in), p_adder3/1(sync_in), p_adder4/1(sync_in)
  in1/1 -> p_adder1/2(in1)
  in2/1 -> p_adder1/3(in2)
  in3/1 -> p_adder1/4(in3)
  in4/1 -> p_adder1/5(in4)
  in5/1 -> p_adder1/6(in5)
  in6/1 -> p_adder1/7(in6)
  in7/1 -> p_adder1/8(in7)
  in8/1 -> p_adder1/9(in8)
  in9/1 -> p_adder1/10(in9)
  in10/1 -> p_adder1/11(in10)
  in11/1 -> p_adder1/12(in11)
  in12/1 -> p_adder1/13(in12)
  in13/1 -> p_adder1/14(in13)
  in14/1 -> p_adder1/15(in14)
  in15/1 -> p_adder1/16(in15)
  in16/1 -> p_adder1/17(in16)
  p_adder1/2(out1) -> p_adder2/2(in1)  "pa_i2_1"
  p_adder1/3(out2) -> p_adder2/3(in2)  "pa_i2_2"
  p_adder1/4(out3) -> p_adder2/4(in3)  "pa_i2_3"
  p_adder1/5(out4) -> p_adder2/5(in4)  "pa_i2_4"
  p_adder1/6(out5) -> p_adder2/6(in5)  "pa_i2_5"
  p_adder1/7(out6) -> p_adder2/7(in6)  "pa_i2_6"
  p_adder1/8(out7) -> p_adder2/8(in7)  "pa_i2_7"
  p_adder1/9(out8) -> p_adder2/9(in8)  "pa_i2_8"
  p_adder1/10(out9) -> p_adder2/10(in9)  "pa_i2_9"
  p_adder1/11(out10) -> p_adder2/11(in10)  "pa_i2_10"
  p_adder1/12(out11) -> p_adder2/12(in11)  "pa_i2_11"
  p_adder1/13(out12) -> p_adder2/13(in12)  "pa_i2_12"
  p_adder1/14(out13) -> p_adder2/14(in13)  "pa_i2_13"
  p_adder1/15(out14) -> p_adder2/15(in14)  "pa_i2_14"
  p_adder1/16(out15) -> p_adder2/16(in15)  "pa_i2_15"
  p_adder1/17(out16) -> p_adder2/17(in16)  "pa_i2_16"
  p_adder2/2(out1) -> p_adder3/2(in1)  "pa_i3_1"
  p_adder2/3(out2) -> p_adder3/3(in2)  "pa_i3_2"
  p_adder2/4(out3) -> p_adder3/4(in3)  "pa_i3_3"
  p_adder2/5(out4) -> p_adder3/5(in4)  "pa_i3_4"
  p_adder2/6(out5) -> p_adder3/6(in5)  "pa_i3_5"
  p_adder2/7(out6) -> p_adder3/7(in6)  "pa_i3_6"
  p_adder2/8(out7) -> p_adder3/8(in7)  "pa_i3_7"
  p_adder2/9(out8) -> p_adder3/9(in8)  "pa_i3_8"
  p_adder2/10(out9) -> p_adder3/10(in9)  "pa_i3_9"
  p_adder2/11(out10) -> p_adder3/11(in10)  "pa_i3_10"
  p_adder2/12(out11) -> p_adder3/12(in11)  "pa_i3_11"
  p_adder2/13(out12) -> p_adder3/13(in12)  "pa_i3_12"
  p_adder2/14(out13) -> p_adder3/14(in13)  "pa_i3_13"
  p_adder2/15(out14) -> p_adder3/15(in14)  "pa_i3_14"
  p_adder2/16(out15) -> p_adder3/16(in15)  "pa_i3_15"
  p_adder2/17(out16) -> p_adder3/17(in16)  "pa_i3_16"
  p_adder3/2(out1) -> p_adder4/2(in1)  "pa_i4_1"
  p_adder3/3(out2) -> p_adder4/3(in2)  "pa_i4_2"
  p_adder3/4(out3) -> p_adder4/4(in3)  "pa_i4_3"
  p_adder3/5(out4) -> p_adder4/5(in4)  "pa_i4_4"
  p_adder3/6(out5) -> p_adder4/6(in5)  "pa_i4_5"
  p_adder3/7(out6) -> p_adder4/7(in6)  "pa_i4_6"
  p_adder3/8(out7) -> p_adder4/8(in7)  "pa_i4_7"
  p_adder3/9(out8) -> p_adder4/9(in8)  "pa_i4_8"
  p_adder3/10(out9) -> p_adder4/10(in9)  "pa_i4_9"
  p_adder3/11(out10) -> p_adder4/11(in10)  "pa_i4_10"
  p_adder3/12(out11) -> p_adder4/12(in11)  "pa_i4_11"
  p_adder3/13(out12) -> p_adder4/13(in12)  "pa_i4_12"
  p_adder3/14(out13) -> p_adder4/14(in13)  "pa_i4_13"
  p_adder3/15(out14) -> p_adder4/15(in14)  "pa_i4_14"
  p_adder3/16(out15) -> p_adder4/16(in15)  "pa_i4_15"
  p_adder3/17(out16) -> p_adder4/17(in16)  "pa_i4_16"
  p_adder4/3(out2) -> out1/1  "pa_i5_2"
  p_adder4/5(out4) -> out2/1  "pa_i5_4"
  p_adder4/7(out6) -> out3/1  "pa_i5_6"
  p_adder4/9(out8) -> out4/1  "pa_i5_8"
  p_adder4/11(out10) -> out5/1  "pa_i5_10"
  p_adder4/13(out12) -> out6/1  "pa_i5_12"
  p_adder4/15(out14) -> out7/1  "pa_i5_14"
  p_adder4/17(out16) -> out8/1  "pa_i5_16"
  p_adder4/1(sync_out) -> sync_out/1  "sync_in5"

== system cichbcic_core/cic_pow2_1/Stage2_dec2 ==
  in1 : Inport
  in2 : Inport  Port=2
  in3 : Inport  Port=3
  in4 : Inport  Port=4
  in5 : Inport  Port=5
  in6 : Inport  Port=6
  in7 : Inport  Port=7
  in8 : Inport  Port=8
  sync_in : Inport  Port=9
  p_adder1 : Subsystem
      settings: AttributesFormatString=|
      | Accumulation Length = 2
      | Add Latency = 1
      | Delay Length =1
  p_adder2 : Subsystem
      settings: AttributesFormatString=|
      | Accumulation Length = 2
      | Add Latency = 1
      | Delay Length =1
  p_adder3 : Subsystem
      settings: AttributesFormatString=|
      | Accumulation Length = 2
      | Add Latency = 1
      | Delay Length =1
  p_adder4 : Subsystem
      settings: AttributesFormatString=|
      | Accumulation Length = 2
      | Add Latency = 1
      | Delay Length =1
  out1 : Outport
  out2 : Outport  Port=2
  out3 : Outport  Port=3
  out4 : Outport  Port=4
  sync_out : Outport  Port=5
  wires:
  sync_in/1 -> p_adder1/1(sync_in), p_adder2/1(sync_in), p_adder3/1(sync_in), p_adder4/1(sync_in)
  in1/1 -> p_adder1/2(in1)
  in2/1 -> p_adder1/3(in2)
  in3/1 -> p_adder1/4(in3)
  in4/1 -> p_adder1/5(in4)
  in5/1 -> p_adder1/6(in5)
  in6/1 -> p_adder1/7(in6)
  in7/1 -> p_adder1/8(in7)
  in8/1 -> p_adder1/9(in8)
  p_adder1/2(out1) -> p_adder2/2(in1)  "pa_i2_1"
  p_adder1/3(out2) -> p_adder2/3(in2)  "pa_i2_2"
  p_adder1/4(out3) -> p_adder2/4(in3)  "pa_i2_3"
  p_adder1/5(out4) -> p_adder2/5(in4)  "pa_i2_4"
  p_adder1/6(out5) -> p_adder2/6(in5)  "pa_i2_5"
  p_adder1/7(out6) -> p_adder2/7(in6)  "pa_i2_6"
  p_adder1/8(out7) -> p_adder2/8(in7)  "pa_i2_7"
  p_adder1/9(out8) -> p_adder2/9(in8)  "pa_i2_8"
  p_adder2/2(out1) -> p_adder3/2(in1)  "pa_i3_1"
  p_adder2/3(out2) -> p_adder3/3(in2)  "pa_i3_2"
  p_adder2/4(out3) -> p_adder3/4(in3)  "pa_i3_3"
  p_adder2/5(out4) -> p_adder3/5(in4)  "pa_i3_4"
  p_adder2/6(out5) -> p_adder3/6(in5)  "pa_i3_5"
  p_adder2/7(out6) -> p_adder3/7(in6)  "pa_i3_6"
  p_adder2/8(out7) -> p_adder3/8(in7)  "pa_i3_7"
  p_adder2/9(out8) -> p_adder3/9(in8)  "pa_i3_8"
  p_adder3/2(out1) -> p_adder4/2(in1)  "pa_i4_1"
  p_adder3/3(out2) -> p_adder4/3(in2)  "pa_i4_2"
  p_adder3/4(out3) -> p_adder4/4(in3)  "pa_i4_3"
  p_adder3/5(out4) -> p_adder4/5(in4)  "pa_i4_4"
  p_adder3/6(out5) -> p_adder4/6(in5)  "pa_i4_5"
  p_adder3/7(out6) -> p_adder4/7(in6)  "pa_i4_6"
  p_adder3/8(out7) -> p_adder4/8(in7)  "pa_i4_7"
  p_adder3/9(out8) -> p_adder4/9(in8)  "pa_i4_8"
  p_adder4/3(out2) -> out1/1  "pa_i5_2"
  p_adder4/5(out4) -> out2/1  "pa_i5_4"
  p_adder4/7(out6) -> out3/1  "pa_i5_6"
  p_adder4/9(out8) -> out4/1  "pa_i5_8"
  p_adder4/1(sync_out) -> sync_out/1  "sync_in5"

== system cichbcic_core/cic_pow2_1/Stage3_dec2 ==
  in1 : Inport
  in2 : Inport  Port=2
  in3 : Inport  Port=3
  in4 : Inport  Port=4
  sync_in : Inport  Port=5
  p_adder1 : Subsystem
      settings: AttributesFormatString=|
      | Accumulation Length = 2
      | Add Latency = 1
      | Delay Length =1
  p_adder2 : Subsystem
      settings: AttributesFormatString=|
      | Accumulation Length = 2
      | Add Latency = 1
      | Delay Length =1
  p_adder3 : Subsystem
      settings: AttributesFormatString=|
      | Accumulation Length = 2
      | Add Latency = 1
      | Delay Length =1
  p_adder4 : Subsystem
      settings: AttributesFormatString=|
      | Accumulation Length = 2
      | Add Latency = 1
      | Delay Length =1
  out1 : Outport
  out2 : Outport  Port=2
  sync_out : Outport  Port=3
  wires:
  sync_in/1 -> p_adder1/1(sync_in), p_adder2/1(sync_in), p_adder3/1(sync_in), p_adder4/1(sync_in)
  in1/1 -> p_adder1/2(in1)
  in2/1 -> p_adder1/3(in2)
  in3/1 -> p_adder1/4(in3)
  in4/1 -> p_adder1/5(in4)
  p_adder1/2(out1) -> p_adder2/2(in1)  "pa_i2_1"
  p_adder1/3(out2) -> p_adder2/3(in2)  "pa_i2_2"
  p_adder1/4(out3) -> p_adder2/4(in3)  "pa_i2_3"
  p_adder1/5(out4) -> p_adder2/5(in4)  "pa_i2_4"
  p_adder2/2(out1) -> p_adder3/2(in1)  "pa_i3_1"
  p_adder2/3(out2) -> p_adder3/3(in2)  "pa_i3_2"
  p_adder2/4(out3) -> p_adder3/4(in3)  "pa_i3_3"
  p_adder2/5(out4) -> p_adder3/5(in4)  "pa_i3_4"
  p_adder3/2(out1) -> p_adder4/2(in1)  "pa_i4_1"
  p_adder3/3(out2) -> p_adder4/3(in2)  "pa_i4_2"
  p_adder3/4(out3) -> p_adder4/4(in3)  "pa_i4_3"
  p_adder3/5(out4) -> p_adder4/5(in4)  "pa_i4_4"
  p_adder4/3(out2) -> out1/1  "pa_i5_2"
  p_adder4/5(out4) -> out2/1  "pa_i5_4"
  p_adder4/1(sync_out) -> sync_out/1  "sync_in5"

== system cichbcic_core/cic_pow2_1/Stage4_dec2 ==
  in1 : Inport
  in2 : Inport  Port=2
  sync_in : Inport  Port=3
  p_adder1 : Subsystem
      settings: AttributesFormatString=|
      | Accumulation Length = 2
      | Add Latency = 1
      | Delay Length =1
  p_adder2 : Subsystem
      settings: AttributesFormatString=|
      | Accumulation Length = 2
      | Add Latency = 1
      | Delay Length =1
  p_adder3 : Subsystem
      settings: AttributesFormatString=|
      | Accumulation Length = 2
      | Add Latency = 1
      | Delay Length =1
  p_adder4 : Subsystem
      settings: AttributesFormatString=|
      | Accumulation Length = 2
      | Add Latency = 1
      | Delay Length =1
  out1 : Outport
  sync_out : Outport  Port=2
  wires:
  sync_in/1 -> p_adder1/1(sync_in), p_adder2/1(sync_in), p_adder3/1(sync_in), p_adder4/1(sync_in)
  in1/1 -> p_adder1/2(in1)
  in2/1 -> p_adder1/3(in2)
  p_adder1/2(out1) -> p_adder2/2(in1)  "pa_i2_1"
  p_adder1/3(out2) -> p_adder2/3(in2)  "pa_i2_2"
  p_adder2/2(out1) -> p_adder3/2(in1)  "pa_i3_1"
  p_adder2/3(out2) -> p_adder3/3(in2)  "pa_i3_2"
  p_adder3/2(out1) -> p_adder4/2(in1)  "pa_i4_1"
  p_adder3/3(out2) -> p_adder4/3(in2)  "pa_i4_2"
  p_adder4/3(out2) -> out1/1  "pa_i5_2"
  p_adder4/1(sync_out) -> sync_out/1  "sync_in5"

== system cichbcic_core/cic_pow2_1/Stage5_dec2 ==
  in : Inport
  sync_in : Inport  Port=2
  Down_sample1 : Subsystem
      settings: AttributesFormatString=|
      | Rate change: 2
      | clock(actualy/effective): 1/1
  adder_tree1 : Subsystem
  adder_tree2 : Subsystem
  adder_tree3 : Subsystem
  adder_tree4 : Subsystem
  delay1_1 : xbsIndex_r4/Delay  rst=off  infoeditControl=Selection of Reset will increase slice count due to use of real FFs and instead of SRLs  en=off  latency=1  dbl_ovrd=off  reg_retiming=off  block_type=delay
  delay2_1 : xbsIndex_r4/Delay  rst=off  infoeditControl=Selection of Reset will increase slice count due to use of real FFs and instead of SRLs  en=off  latency=1  dbl_ovrd=off  reg_retiming=off  block_type=delay
  delay3_1 : xbsIndex_r4/Delay  rst=off  infoeditControl=Selection of Reset will increase slice count due to use of real FFs and instead of SRLs  en=off  latency=1  dbl_ovrd=off  reg_retiming=off  block_type=delay
  delay4_1 : xbsIndex_r4/Delay  rst=off  infoeditControl=Selection of Reset will increase slice count due to use of real FFs and instead of SRLs  en=off  latency=1  dbl_ovrd=off  reg_retiming=off  block_type=delay
  out : Outport
  sync_out : Outport  Port=2
  wires:
  in/1 -> delay1_1/1, adder_tree1/1(sync), adder_tree1/2(din_1)
  delay1_1/1 -> adder_tree1/3(din_2)  "delay_out1_2"
  adder_tree1/2(dout) -> delay2_1/1, adder_tree2/2(din_1)  "delay_in1_1"
  adder_tree1/1(sync_out) -> adder_tree2/1(sync)  "adder_tree_sync_in2"
  delay2_1/1 -> adder_tree2/3(din_2)  "delay_out2_2"
  adder_tree2/2(dout) -> delay3_1/1, adder_tree3/2(din_1)  "delay_in2_1"
  adder_tree2/1(sync_out) -> adder_tree3/1(sync)  "adder_tree_sync_in3"
  delay3_1/1 -> adder_tree3/3(din_2)  "delay_out3_2"
  adder_tree3/2(dout) -> delay4_1/1, adder_tree4/2(din_1)  "delay_in3_1"
  adder_tree3/1(sync_out) -> adder_tree4/1(sync)  "adder_tree_sync_in4"
  delay4_1/1 -> adder_tree4/3(din_2)  "delay_out4_2"
  adder_tree4/2(dout) -> Down_sample1/1(In)  "delay_in4_1"
  sync_in/1 -> Down_sample1/2(sync_in)
  Down_sample1/1(Out) -> out/1
  Down_sample1/2(sync_out) -> sync_out/1

== system cichbcic_core/cic_stage_dec3/Down_sample1 ==
  In : Inport
  sync_in : Inport  Port=2
  Register : xbsIndex_r4/Register  init=0  rst=off  en=on  dbl_ovrd=off  block_type=register
  en_gen : Subsystem
      settings: AttributesFormatString=|
      | hold period: 8
      | explicit clk period:on , input clk period:1
  sync_delay : xbsIndex_r4/Delay  rst=off  infoeditControl=Selection of Reset will increase slice count due to use of real FFs and instead of SRLs  en=off  latency=1  dbl_ovrd=off  reg_retiming=off  block_type=delay
  Out : Outport
  sync_out : Outport  Port=2
  wires:
  sync_in/1 -> en_gen/1(sync_in), sync_delay/1
  In/1 -> Register/1
  en_gen/1(en_out) -> Register/2  "en"
  Register/1 -> Out/1
  sync_delay/1 -> sync_out/1

== system cichbcic_core/cic_stage_dec3/adder_tree1 ==
  sync : Inport
  din_1 : Inport  Port=2
  din_2 : Inport  Port=3
  adder_0 : xbsIndex_r4/AddSub  mode=Addition  use_carryin=off  use_carryout=off  en=off  latency=8  precision=Full  arith_type=Unsigned  n_bits=18  bin_pt=17  quantization="Round  (unbiased: +/- Inf)"  overflow=Saturate  dbl_ovrd=off  use_behavioral_HDL=on  hw_selection=Fabric  pipelined=off  block_type=addsub
  sync_delay : xbsIndex_r4/Delay  rst=off  infoeditControl=Selection of Reset will increase slice count due to use of real FFs and instead of SRLs  en=off  latency=8  dbl_ovrd=off  reg_retiming=off  block_type=delay
  sync_out : Outport
  dout : Outport  Port=2
  wires:
  sync/1 -> sync_delay/1
  sync_delay/1 -> sync_out/1
  din_2/1 -> adder_0/1
  din_1/1 -> adder_0/2
  adder_0/1 -> dout/1

== system cichbcic_core/cic_stage_dec3/adder_tree2 ==
  sync : Inport
  din_1 : Inport  Port=2
  din_2 : Inport  Port=3
  adder_0 : xbsIndex_r4/AddSub  mode=Addition  use_carryin=off  use_carryout=off  en=off  latency=8  precision=Full  arith_type=Unsigned  n_bits=18  bin_pt=17  quantization="Round  (unbiased: +/- Inf)"  overflow=Saturate  dbl_ovrd=off  use_behavioral_HDL=on  hw_selection=Fabric  pipelined=off  block_type=addsub
  sync_delay : xbsIndex_r4/Delay  rst=off  infoeditControl=Selection of Reset will increase slice count due to use of real FFs and instead of SRLs  en=off  latency=8  dbl_ovrd=off  reg_retiming=off  block_type=delay
  sync_out : Outport
  dout : Outport  Port=2
  wires:
  sync/1 -> sync_delay/1
  sync_delay/1 -> sync_out/1
  din_2/1 -> adder_0/1
  din_1/1 -> adder_0/2
  adder_0/1 -> dout/1

== system cichbcic_core/cic_stage_dec3/adder_tree3 ==
  sync : Inport
  din_1 : Inport  Port=2
  din_2 : Inport  Port=3
  adder_0 : xbsIndex_r4/AddSub  mode=Addition  use_carryin=off  use_carryout=off  en=off  latency=8  precision=Full  arith_type=Unsigned  n_bits=18  bin_pt=17  quantization="Round  (unbiased: +/- Inf)"  overflow=Saturate  dbl_ovrd=off  use_behavioral_HDL=on  hw_selection=Fabric  pipelined=off  block_type=addsub
  sync_delay : xbsIndex_r4/Delay  rst=off  infoeditControl=Selection of Reset will increase slice count due to use of real FFs and instead of SRLs  en=off  latency=8  dbl_ovrd=off  reg_retiming=off  block_type=delay
  sync_out : Outport
  dout : Outport  Port=2
  wires:
  sync/1 -> sync_delay/1
  sync_delay/1 -> sync_out/1
  din_2/1 -> adder_0/1
  din_1/1 -> adder_0/2
  adder_0/1 -> dout/1

== system cichbcic_core/cic_stage_dec4/Down_sample1 ==
  In : Inport
  sync_in : Inport  Port=2
  Register : xbsIndex_r4/Register  init=0  rst=off  en=on  dbl_ovrd=off  block_type=register
  en_gen : Subsystem
      settings: AttributesFormatString=|
      | hold period: 4
      | explicit clk period:on , input clk period:1
  sync_delay : xbsIndex_r4/Delay  rst=off  infoeditControl=Selection of Reset will increase slice count due to use of real FFs and instead of SRLs  en=off  latency=1  dbl_ovrd=off  reg_retiming=off  block_type=delay
  Out : Outport
  sync_out : Outport  Port=2
  wires:
  sync_in/1 -> en_gen/1(sync_in), sync_delay/1
  In/1 -> Register/1
  en_gen/1(en_out) -> Register/2  "en"
  Register/1 -> Out/1
  sync_delay/1 -> sync_out/1
